simulink model "mrefrobotarm_previous_y_previous_u_previous_ref_cex_3b"  (R2018b)
settings: Solver=FixedStepAuto  StartTime=0.0  StopTime=20  RelTol=1e-3  AbsTol=1e-6
undefined symbols (not defined in the file or in its folder): cc, options
libraries: neural x462, simulink x2
(part 10 of 18)

== system mrefrobotarm_previous_y_previous_u_previous_ref_cex_3b/5000_epoch/Layer 3/Delays 1 ==
  "p{3}" : Inport  PortDimensions=30
      mask Display: e = 0.06;c1 = [120 230 180]/255;c2 = ([120 230 180]+0)/(256+128);c3 = ([120 230 180]+128)/(256+128);patch([0 1 1 0],[0 0 1 1],c1);patch([0 1 1 1-e 1-e 0+e],[0 0 1 1-e 0+e 0+e],c2);patch([0 0 1 1-e 0+e 0+e],[0 1 1 1-e 1-e 0+e],c3);plot([0 1 1 0 0],[0 0 1 1 0]);
  mux : Mux  Inputs=1
      mask Display: e = 0.06;c1 = [120 150 230]/255;c2 = ([120 150 230]+0)/383;c3 = ([120 150 230]+128)/383;patch([0 1 1 0],[0 0 1 1],c1);patch([0 1 1 1-e 1-e 0+e],[0 0 1 1-e 0+e 0+e],c2);patch([0 0 1 1-e 0+e 0+e],[0 1 1 1-e 1-e 0+e],c3);plot([0 1 1 0 0],[0 0 1 1 0]);disp('Mux')
  "pd{3,2}" : Outport
      mask Display: e = 0.06;c1 = [120 230 180]/255;c2 = ([120 230 180]+0)/(256+128);c3 = ([120 230 180]+128)/(256+128);patch([0 1 1 0],[0 0 1 1],c1);patch([0 1 1 1-e 1-e 0+e],[0 0 1 1-e 0+e 0+e],c2);patch([0 0 1 1-e 0+e 0+e],[0 1 1 1-e 1-e 0+e],c3);plot([0 1 1 0 0],[0 0 1 1 0]);
  wires:
  "p{3}"/1 -> mux/1
  mux/1 -> "pd{3,2}"/1

== system mrefrobotarm_previous_y_previous_u_previous_ref_cex_3b/5000_epoch/Layer 3/LW{3,2} ==
  "ad{3,2}" : Inport  PortDimensions=30
      mask Display: e = 0.06;c1 = [120 230 180]/255;c2 = ([120 230 180]+0)/(256+128);c3 = ([120 230 180]+128)/(256+128);patch([0 1 1 0],[0 0 1 1],c1);patch([0 1 1 1-e 1-e 0+e],[0 0 1 1-e 0+e 0+e],c2);patch([0 0 1 1-e 0+e 0+e],[0 1 1 1-e 1-e 0+e],c3);plot([0 1 1 0 0],[0 0 1 1 0]);
  "IW{3,2}(1,:)'" : Constant  Value=[0.07120769791695548411869509664029465056955814361572265625;0.293957514102999251104364475395414046943187713623046875;-0.102217807051302178589224922689027152955532073974609375;-0.4928214954328120622761844060732983052730560302734375;-0.6859335778553450335692787120933644473552703857421875;0.10215887737343372354548165503729251213371753692626953125;0.1810653784287956924448081963419099338352680206298828125;0.278110114235700145446372744117979891598224639892578125;0.165277512488851197058892239510896615684032440185546875;-0.58534311597175092689582243110635317862033843994140625;0.1463336102721248532798625774375977925956249237060546875;-0.134800489251362842768600103227072395384311676025390625;-0.8834099653862776957424784995964728295803070068359375;-0.402877151040579140062192209370550699532032012939453125;-0.9904548377251851665192816653870977461338043212890625;0.07516141105989652959618041450085001997649669647216796875;0.256462278810463517597639793166308663785457611083984375;0.133927541929137861043130897087394259870052337646484375;0.937187293052101910717510691029019653797149658203125;0.344579518523550454300874434920842759311199188232421875;-0.12401331514423587221163103322396636940538883209228515625;-0.7653357924133674661248960546799935400485992431640625;0.6146453163710081657455930326250381767749786376953125;0.2201364801288865080675094532125513069331645965576171875;-0.86449912385295324401823791049537248909473419189453125;-0.543957967972903855269350970047526061534881591796875;0.290966307623606146304240382960415445268154144287109375;0.10258338058370508605321447248570621013641357421875;0.100254156699624397131032083052559755742549896240234375;0.34509165546467002183561589845339767634868621826171875]
      mask Display: e = 0.06;c1 = [120 150 230]/255;c2 = ([120 150 230]+0)/383;c3 = ([120 150 230]+128)/383;patch([0 1 1 0],[0 0 1 1],c1);patch([0 1 1 1-e 1-e 0+e],[0 0 1 1-e 0+e 0+e],c2);patch([0 0 1 1-e 0+e 0+e],[0 1 1 1-e 1-e 0+e],c3);plot([0 1 1 0 0],[0 0 1 1 0]);disp('weights');
  Mux : Mux  Inputs=1
      mask Display: e = 0.06;c1 = [120 150 230]/255;c2 = ([120 150 230]+0)/383;c3 = ([120 150 230]+128)/383;patch([0 1 1 0],[0 0 1 1],c1);patch([0 1 1 1-e 1-e 0+e],[0 0 1 1-e 0+e 0+e],c2);patch([0 0 1 1-e 0+e 0+e],[0 1 1 1-e 1-e 0+e],c3);plot([0 1 1 0 0],[0 0 1 1 0]);disp('Mux');
  dotprod1 : neural/Weight Functions/dotprod
  "lz{3,2}" : Outport
      mask Display: e = 0.06;c1 = [120 230 180]/255;c2 = ([120 230 180]+0)/(256+128);c3 = ([120 230 180]+128)/(256+128);patch([0 1 1 0],[0 0 1 1],c1);patch([0 1 1 1-e 1-e 0+e],[0 0 1 1-e 0+e 0+e],c2);patch([0 0 1 1-e 0+e 0+e],[0 1 1 1-e 1-e 0+e],c3);plot([0 1 1 0 0],[0 0 1 1 0]);
  wires:
  "IW{3,2}(1,:)'"/1 -> dotprod1/1
  "ad{3,2}"/1 -> dotprod1/2
  dotprod1/1 -> Mux/1
  Mux/1 -> "lz{3,2}"/1

== system mrefrobotarm_previous_y_previous_u_previous_ref_cex_3b/cex_m1/Layer 1/Delays 1 ==
  "p{1}" : Inport  PortDimensions=10
      mask Display: e = 0.06;c1 = [120 230 180]/255;c2 = ([120 230 180]+0)/(256+128);c3 = ([120 230 180]+128)/(256+128);patch([0 1 1 0],[0 0 1 1],c1);patch([0 1 1 1-e 1-e 0+e],[0 0 1 1-e 0+e 0+e],c2);patch([0 0 1 1-e 0+e 0+e],[0 1 1 1-e 1-e 0+e],c3);plot([0 1 1 0 0],[0 0 1 1 0]);
  mux : Mux  Inputs=1
      mask Display: e = 0.06;c1 = [120 150 230]/255;c2 = ([120 150 230]+0)/383;c3 = ([120 150 230]+128)/383;patch([0 1 1 0],[0 0 1 1],c1);patch([0 1 1 1-e 1-e 0+e],[0 0 1 1-e 0+e 0+e],c2);patch([0 0 1 1-e 0+e 0+e],[0 1 1 1-e 1-e 0+e],c3);plot([0 1 1 0 0],[0 0 1 1 0]);disp('Mux')
  "pd{1,1}" : Outport
      mask Display: e = 0.06;c1 = [120 230 180]/255;c2 = ([120 230 180]+0)/(256+128);c3 = ([120 230 180]+128)/(256+128);patch([0 1 1 0],[0 0 1 1],c1);patch([0 1 1 1-e 1-e 0+e],[0 0 1 1-e 0+e 0+e],c2);patch([0 0 1 1-e 0+e 0+e],[0 1 1 1-e 1-e 0+e],c3);plot([0 1 1 0 0],[0 0 1 1 0]);
  wires:
  "p{1}"/1 -> mux/1
  mux/1 -> "pd{1,1}"/1

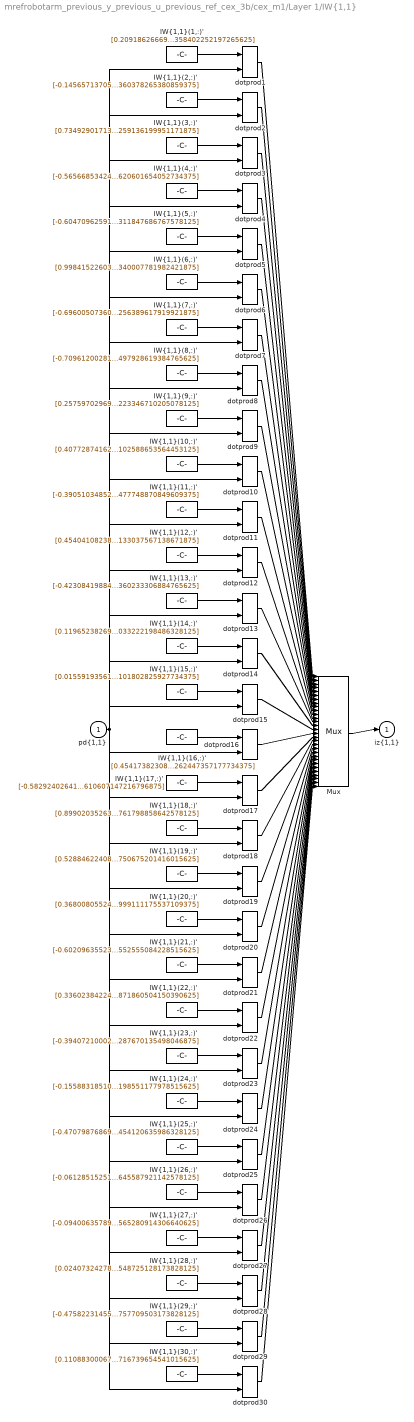
== system mrefrobotarm_previous_y_previous_u_previous_ref_cex_3b/cex_m1/Layer 1/IW{1,1} ==
  "pd{1,1}" : Inport  PortDimensions=10
      mask Display: e = 0.06;c1 = [120 230 180]/255;c2 = ([120 230 180]+0)/(256+128);c3 = ([120 230 180]+128)/(256+128);patch([0 1 1 0],[0 0 1 1],c1);patch([0 1 1 1-e 1-e 0+e],[0 0 1 1-e 0+e 0+e],c2);patch([0 0 1 1-e 0+e 0+e],[0 1 1 1-e 1-e 0+e],c3);plot([0 1 1 0 0],[0 0 1 1 0]);
  "IW{1,1}(1,:)'" : Constant  Value=[0.2091862666929468483889564822675311006605625152587890625;0.55963348740756568844290086417458951473236083984375;0.0245060466286013134418197978448006324470043182373046875;0.2178988291207533400939411194485728628933429718017578125;-0.26749825460170051361075138629530556499958038330078125;0.66511017670048844241392771436949260532855987548828125;-0.89337790569789710115600200879271142184734344482421875;-0.68360390444573138069017659290693700313568115234375;-0.01825482404689289517296657550105010159313678741455078125;-0.88702631490236660827264358886168338358402252197265625]
      mask Display: e = 0.06;c1 = [120 150 230]/255;c2 = ([120 150 230]+0)/383;c3 = ([120 150 230]+128)/383;patch([0 1 1 0],[0 0 1 1],c1);patch([0 1 1 1-e 1-e 0+e],[0 0 1 1-e 0+e 0+e],c2);patch([0 0 1 1-e 0+e 0+e],[0 1 1 1-e 1-e 0+e],c3);plot([0 1 1 0 0],[0 0 1 1 0]);disp('Weights');
  "IW{1,1}(10,:)'" : Constant  Value=[0.407728741626480040149971273422124795615673065185546875;-1.09823873025257778834884447860531508922576904296875;0.29259795109139952185017818919732235372066497802734375;0.345075553219635511315033227219828404486179351806640625;0.6166793772066860856995162976090796291828155517578125;-0.53009927483939034420501457134378142654895782470703125;-0.29346314878497825606729065839317627251148223876953125;0.388864437565445031363964289994328282773494720458984375;-0.022174851916459244194346211997981299646198749542236328125;0.82461100280284871377745048448559828102588653564453125]
      mask Display: e = 0.06;c1 = [120 150 230]/255;c2 = ([120 150 230]+0)/383;c3 = ([120 150 230]+128)/383;patch([0 1 1 0],[0 0 1 1],c1);patch([0 1 1 1-e 1-e 0+e],[0 0 1 1-e 0+e 0+e],c2);patch([0 0 1 1-e 0+e 0+e],[0 1 1 1-e 1-e 0+e],c3);plot([0 1 1 0 0],[0 0 1 1 0]);disp('Weights');
  "IW{1,1}(11,:)'" : Constant  Value=[-0.390510348523106454177167279340210370719432830810546875;0.280930746398683039988242171602905727922916412353515625;0.08856122912073373376617979602087871171534061431884765625;0.0183926105937365184928022898702693055383861064910888671875;-0.08511188285763936212102720446637249551713466644287109375;-1.2933297714879312678704081918112933635711669921875;0.20346443800545410685032265973859466612339019775390625;0.59287238698671185233024516492150723934173583984375;-0.51455352543008781029953979668789543211460113525390625;0.2082980484226676087811114257419831119477748870849609375]
      mask Display: e = 0.06;c1 = [120 150 230]/255;c2 = ([120 150 230]+0)/383;c3 = ([120 150 230]+128)/383;patch([0 1 1 0],[0 0 1 1],c1);patch([0 1 1 1-e 1-e 0+e],[0 0 1 1-e 0+e 0+e],c2);patch([0 0 1 1-e 0+e 0+e],[0 1 1 1-e 1-e 0+e],c3);plot([0 1 1 0 0],[0 0 1 1 0]);disp('Weights');
  "IW{1,1}(12,:)'" : Constant  Value=[0.454041082380829352782569685587077401578426361083984375;-0.108216191956810703356239855565945617854595184326171875;-0.50433758821169483166357849768246524035930633544921875;0.34650587412748390381267427073908038437366485595703125;0.51861097707927428235308298098971135914325714111328125;-0.75606936535445401492694372791447676718235015869140625;-0.474625539848971766954122131210169754922389984130859375;0.062468383097865766429013234528611064888536930084228515625;0.55093241527519953848468503565527498722076416015625;-0.620778109366568298099764433573000133037567138671875]
      mask Display: e = 0.06;c1 = [120 150 230]/255;c2 = ([120 150 230]+0)/383;c3 = ([120 150 230]+128)/383;patch([0 1 1 0],[0 0 1 1],c1);patch([0 1 1 1-e 1-e 0+e],[0 0 1 1-e 0+e 0+e],c2);patch([0 0 1 1-e 0+e 0+e],[0 1 1 1-e 1-e 0+e],c3);plot([0 1 1 0 0],[0 0 1 1 0]);disp('Weights');
  "IW{1,1}(13,:)'" : Constant  Value=[-0.423084198848980796991980923849041573703289031982421875;-0.53304476363188302290296860519447363913059234619140625;-0.565627651828932709321406946401111781597137451171875;0.417830660461573299979676221482804976403713226318359375;0.60632158873281605249161430037929676473140716552734375;0.9207074477285381863822522063856013119220733642578125;-0.95014294107361652041987554184743203222751617431640625;0.0424423038346196934700316205635317601263523101806640625;-0.1643176448134923972599352737233857624232769012451171875;1.0022089026863645333520480562583543360233306884765625]
      mask Display: e = 0.06;c1 = [120 150 230]/255;c2 = ([120 150 230]+0)/383;c3 = ([120 150 230]+128)/383;patch([0 1 1 0],[0 0 1 1],c1);patch([0 1 1 1-e 1-e 0+e],[0 0 1 1-e 0+e 0+e],c2);patch([0 0 1 1-e 0+e 0+e],[0 1 1 1-e 1-e 0+e],c3);plot([0 1 1 0 0],[0 0 1 1 0]);disp('Weights');
  "IW{1,1}(14,:)'" : Constant  Value=[0.1196523826915620869471013065776787698268890380859375;0.203688796664640181521832573707797564566135406494140625;-0.0471376839766617095062173348196665756404399871826171875;0.474187802455269091783662815942079760134220123291015625;-1.019539841234085475463189141009934246540069580078125;0.31052365757284672298510486143641173839569091796875;-0.7583308622335831472582867718301713466644287109375;0.2650487385605939660848662242642603814601898193359375;0.05457125001518541018707963985434616915881633758544921875;-0.0952582112585181051134242125044693239033222198486328125]
      mask Display: e = 0.06;c1 = [120 150 230]/255;c2 = ([120 150 230]+0)/383;c3 = ([120 150 230]+128)/383;patch([0 1 1 0],[0 0 1 1],c1);patch([0 1 1 1-e 1-e 0+e],[0 0 1 1-e 0+e 0+e],c2);patch([0 0 1 1-e 0+e 0+e],[0 1 1 1-e 1-e 0+e],c3);plot([0 1 1 0 0],[0 0 1 1 0]);disp('Weights');
  "IW{1,1}(15,:)'" : Constant  Value=[0.0155919356143503391731730545188838732428848743438720703125;0.269803619589356113994682573320460505783557891845703125;0.147051842439241242654901498099206946790218353271484375;-0.7745868105897117938951623727916739881038665771484375;1.2903168482513975856562638000468723475933074951171875;-0.4201312277855315802099767097388394176959991455078125;-0.226047840789400933392272463606786914169788360595703125;-0.72869256085332534400578197164577431976795196533203125;-0.40668314497398128093408331551472656428813934326171875;-0.74033295636701035302706941365613602101802825927734375]
      mask Display: e = 0.06;c1 = [120 150 230]/255;c2 = ([120 150 230]+0)/383;c3 = ([120 150 230]+128)/383;patch([0 1 1 0],[0 0 1 1],c1);patch([0 1 1 1-e 1-e 0+e],[0 0 1 1-e 0+e 0+e],c2);patch([0 0 1 1-e 0+e 0+e],[0 1 1 1-e 1-e 0+e],c3);plot([0 1 1 0 0],[0 0 1 1 0]);disp('Weights');
  "IW{1,1}(16,:)'" : Constant  Value=[0.454173823086521932790304845184436999261379241943359375;-0.800364086576109468040840511093847453594207763671875;0.280125159478748997354813354832003824412822723388671875;-0.8182209528732153902552681756787933409214019775390625;1.8090173847658237438196238144882954657077789306640625;0.5022417744867786471019144300953485071659088134765625;-1.169078109472902138321614984306506812572479248046875;-0.5998812716593977523160674536484293639659881591796875;-0.0400917281417088322559294510938343591988086700439453125;0.331029591208813422920087532475008629262447357177734375]
      mask Display: e = 0.06;c1 = [120 150 230]/255;c2 = ([120 150 230]+0)/383;c3 = ([120 150 230]+128)/383;patch([0 1 1 0],[0 0 1 1],c1);patch([0 1 1 1-e 1-e 0+e],[0 0 1 1-e 0+e 0+e],c2);patch([0 0 1 1-e 0+e 0+e],[0 1 1 1-e 1-e 0+e],c3);plot([0 1 1 0 0],[0 0 1 1 0]);disp('Weights');
  "IW{1,1}(17,:)'" : Constant  Value=[-0.5829240264146486882879116819822229444980621337890625;0.98504904866951614739178921809070743620395660400390625;-0.2542168950231253887750426656566560268402099609375;0.509425718623048862099267353187315165996551513671875;0.71815029183283496383438659904641099274158477783203125;-0.97456899966675691882045384772936813533306121826171875;-0.1697229391253351205026689285659813322126865386962890625;0.1636748206886007028781904182324069552123546600341796875;0.255098819940770826786291536336648277938365936279296875;-0.5024198673275594995146775545435957610607147216796875]
      mask Display: e = 0.06;c1 = [120 150 230]/255;c2 = ([120 150 230]+0)/383;c3 = ([120 150 230]+128)/383;patch([0 1 1 0],[0 0 1 1],c1);patch([0 1 1 1-e 1-e 0+e],[0 0 1 1-e 0+e 0+e],c2);patch([0 0 1 1-e 0+e 0+e],[0 1 1 1-e 1-e 0+e],c3);plot([0 1 1 0 0],[0 0 1 1 0]);disp('Weights');
  "IW{1,1}(18,:)'" : Constant  Value=[0.8990203526391773447556943210656754672527313232421875;-0.471686438787703832264952552577597089111804962158203125;-0.892914200230652710388312698341906070709228515625;-0.07007749122282362630453889096315833739936351776123046875;0.1677092178341874906255526411769096739590167999267578125;0.279705943970333492654134488475392572581768035888671875;0.1259915830780845846792459497009986080229282379150390625;-0.6503287762770748603458059733384288847446441650390625;-0.6518112623153899942707312220591120421886444091796875;-0.56845180521082661062592933376436121761798858642578125]
      mask Display: e = 0.06;c1 = [120 150 230]/255;c2 = ([120 150 230]+0)/383;c3 = ([120 150 230]+128)/383;patch([0 1 1 0],[0 0 1 1],c1);patch([0 1 1 1-e 1-e 0+e],[0 0 1 1-e 0+e 0+e],c2);patch([0 0 1 1-e 0+e 0+e],[0 1 1 1-e 1-e 0+e],c3);plot([0 1 1 0 0],[0 0 1 1 0]);disp('Weights');
  "IW{1,1}(19,:)'" : Constant  Value=[0.52884622408495352008372947238967753946781158447265625;0.34089759980611511469561492049251683056354522705078125;-0.448295411265493048968977518597966991364955902099609375;0.7316745664736530319061103000422008335590362548828125;0.01119555977979982096248701139984405017457902431488037109375;-0.87063334773666412047532503493130207061767578125;0.7710191192510136293236655546934343874454498291015625;0.70429711176034748287833053836948238313198089599609375;0.53710793489006924961159938902710564434528350830078125;-0.54623479056526580421859762282110750675201416015625]
      mask Display: e = 0.06;c1 = [120 150 230]/255;c2 = ([120 150 230]+0)/383;c3 = ([120 150 230]+128)/383;patch([0 1 1 0],[0 0 1 1],c1);patch([0 1 1 1-e 1-e 0+e],[0 0 1 1-e 0+e 0+e],c2);patch([0 0 1 1-e 0+e 0+e],[0 1 1 1-e 1-e 0+e],c3);plot([0 1 1 0 0],[0 0 1 1 0]);disp('Weights');
  "IW{1,1}(2,:)'" : Constant  Value=[-0.14565713705002547584399508195929229259490966796875;0.92722440151880702874365169918746687471866607666015625;-0.58041816336865037495584829230210743844509124755859375;0.327140195131600031164254005489055998623371124267578125;-0.929859979711404438518229653709568083286285400390625;-0.74872830114199062645496951517998240888118743896484375;0.385940683264537398589055783304502256214618682861328125;0.6107778553311418168192403754801489412784576416015625;0.75481290789782995442891433413024060428142547607421875;-0.235879183916507084717295583686791360378265380859375]
      mask Display: e = 0.06;c1 = [120 150 230]/255;c2 = ([120 150 230]+0)/383;c3 = ([120 150 230]+128)/383;patch([0 1 1 0],[0 0 1 1],c1);patch([0 1 1 1-e 1-e 0+e],[0 0 1 1-e 0+e 0+e],c2);patch([0 0 1 1-e 0+e 0+e],[0 1 1 1-e 1-e 0+e],c3);plot([0 1 1 0 0],[0 0 1 1 0]);disp('Weights');
  "IW{1,1}(20,:)'" : Constant  Value=[0.368008055243381371202104901385609991848468780517578125;-0.002192585139888168256627754004739472293294966220855712890625;0.0563330526990998559089263153509818948805332183837890625;0.352091098525261270157926674073678441345691680908203125;0.385736390538022166918352695574867539107799530029296875;-0.247630614263226467297585031701601110398769378662109375;0.58477909697959418178214718864182941615581512451171875;0.1562187305741310205942085076458170078694820404052734375;0.82360238974781430076888000257895328104496002197265625;-0.476230943299036757476727643734193406999111175537109375]
      mask Display: e = 0.06;c1 = [120 150 230]/255;c2 = ([120 150 230]+0)/383;c3 = ([120 150 230]+128)/383;patch([0 1 1 0],[0 0 1 1],c1);patch([0 1 1 1-e 1-e 0+e],[0 0 1 1-e 0+e 0+e],c2);patch([0 0 1 1-e 0+e 0+e],[0 1 1 1-e 1-e 0+e],c3);plot([0 1 1 0 0],[0 0 1 1 0]);disp('Weights');
  "IW{1,1}(21,:)'" : Constant  Value=[-0.60209635523566762405067720465012826025485992431640625;-0.0716463435268997195226603480477933771908283233642578125;0.271658003646719325985259274602867662906646728515625;-0.5095289852754951720470444342936389148235321044921875;0.15508802660567211351150262998999096453189849853515625;-0.400285938688359710369013555464334785938262939453125;0.147605255136038504559792272630147635936737060546875;-0.0248094629809944879073047019346631714142858982086181640625;-1.0605743434036065675485360770835541188716888427734375;0.69405662206880069931003163219429552555084228515625]
      mask Display: e = 0.06;c1 = [120 150 230]/255;c2 = ([120 150 230]+0)/383;c3 = ([120 150 230]+128)/383;patch([0 1 1 0],[0 0 1 1],c1);patch([0 1 1 1-e 1-e 0+e],[0 0 1 1-e 0+e 0+e],c2);patch([0 0 1 1-e 0+e 0+e],[0 1 1 1-e 1-e 0+e],c3);plot([0 1 1 0 0],[0 0 1 1 0]);disp('Weights');
  "IW{1,1}(22,:)'" : Constant  Value=[0.33602384224934456202760202359058894217014312744140625;0.316854130288579616259170279590762220323085784912109375;-0.37857291065639475657889079229789786040782928466796875;0.85810737036911899355828836633008904755115509033203125;-1.04134819912401699326665038825012743473052978515625;0.348267620019931722907813309575431048870086669921875;0.68524259659312536374642377268173731863498687744140625;0.68116189574731322853295978347887285053730010986328125;0.053809239235190174654999140102518140338361263275146484375;0.071470638811097553233508961056941188871860504150390625]
      mask Display: e = 0.06;c1 = [120 150 230]/255;c2 = ([120 150 230]+0)/383;c3 = ([120 150 230]+128)/383;patch([0 1 1 0],[0 0 1 1],c1);patch([0 1 1 1-e 1-e 0+e],[0 0 1 1-e 0+e 0+e],c2);patch([0 0 1 1-e 0+e 0+e],[0 1 1 1-e 1-e 0+e],c3);plot([0 1 1 0 0],[0 0 1 1 0]);disp('Weights');
  "IW{1,1}(23,:)'" : Constant  Value=[-0.394072100026185534460410053725354373455047607421875;1.11211173361084636468376629636622965335845947265625;-0.320213097632206455944725576046039350330829620361328125;0.50688355043374588859705909271724522113800048828125;-0.0849486697110029276291953692634706385433673858642578125;-0.96291306803094289801236982384580187499523162841796875;-0.377668560200759617639931775556760840117931365966796875;0.0946944889176795923102503138579777441918849945068359375;-0.32170494180800834893574347006506286561489105224609375;-0.5240786394310272822139040727051906287670135498046875]
      mask Display: e = 0.06;c1 = [120 150 230]/255;c2 = ([120 150 230]+0)/383;c3 = ([120 150 230]+128)/383;patch([0 1 1 0],[0 0 1 1],c1);patch([0 1 1 1-e 1-e 0+e],[0 0 1 1-e 0+e 0+e],c2);patch([0 0 1 1-e 0+e 0+e],[0 1 1 1-e 1-e 0+e],c3);plot([0 1 1 0 0],[0 0 1 1 0]);disp('Weights');
  "IW{1,1}(24,:)'" : Constant  Value=[-0.1558831851007405067122135733370669186115264892578125;0.844094882972143079058469083975069224834442138671875;-0.162691690832094337793023441918194293975830078125;0.016237577929413653243795323533049668185412883758544921875;-1.1894624225200374212363385595381259918212890625;0.82329478893758312185724435039446689188480377197265625;0.1589582061303255466899742032182984985411167144775390625;0.6871248504549163360621832907781936228275299072265625;0.58317539415476515873848484261543489992618560791015625;0.74057525253661238284763612682581879198551177978515625]
      mask Display: e = 0.06;c1 = [120 150 230]/255;c2 = ([120 150 230]+0)/383;c3 = ([120 150 230]+128)/383;patch([0 1 1 0],[0 0 1 1],c1);patch([0 1 1 1-e 1-e 0+e],[0 0 1 1-e 0+e 0+e],c2);patch([0 0 1 1-e 0+e 0+e],[0 1 1 1-e 1-e 0+e],c3);plot([0 1 1 0 0],[0 0 1 1 0]);disp('Weights');
  "IW{1,1}(25,:)'" : Constant  Value=[-0.470798768696179925630218576770857907831668853759765625;0.5088878241581531458592735361889936029911041259765625;-0.611957297078266737599960833904333412647247314453125;-0.2312082540432938981833643765639862976968288421630859375;0.83570652856447136258566388278268277645111083984375;-0.118154714584164877155814110665232874453067779541015625;0.35551510319171286678141541415243409574031829833984375;-0.8469436595621215868590070385835133492946624755859375;-0.59937255562654867535599123584688641130924224853515625;0.66725706794129735488496635298361070454120635986328125]
      mask Display: e = 0.06;c1 = [120 150 230]/255;c2 = ([120 150 230]+0)/383;c3 = ([120 150 230]+128)/383;patch([0 1 1 0],[0 0 1 1],c1);patch([0 1 1 1-e 1-e 0+e],[0 0 1 1-e 0+e 0+e],c2);patch([0 0 1 1-e 0+e 0+e],[0 1 1 1-e 1-e 0+e],c3);plot([0 1 1 0 0],[0 0 1 1 0]);disp('Weights');
  "IW{1,1}(26,:)'" : Constant  Value=[-0.061285152510976374784501530257330159656703472137451171875;-0.347078272120007691459164789193891920149326324462890625;0.79386039204182001771670229572919197380542755126953125;-0.1920622851114592577470574497056077234447002410888671875;-0.267201831261956013197078618759405799210071563720703125;0.7955336654175482191675428111921064555644989013671875;-0.52745915842468471534942864309414289891719818115234375;-0.451184299445789249727312153481761924922466278076171875;-0.70192132144373264868164596919086761772632598876953125;-0.01597233306397490004702177657236461527645587921142578125]
      mask Display: e = 0.06;c1 = [120 150 230]/255;c2 = ([120 150 230]+0)/383;c3 = ([120 150 230]+128)/383;patch([0 1 1 0],[0 0 1 1],c1);patch([0 1 1 1-e 1-e 0+e],[0 0 1 1-e 0+e 0+e],c2);patch([0 0 1 1-e 0+e 0+e],[0 1 1 1-e 1-e 0+e],c3);plot([0 1 1 0 0],[0 0 1 1 0]);disp('Weights');
  "IW{1,1}(27,:)'" : Constant  Value=[-0.094006357895163372706548443602514453232288360595703125;0.50258758717796070403238672952284105122089385986328125;-0.3250885797258644682727890540263615548610687255859375;0.6097656985874697621596851604408584535121917724609375;-0.768193443515825524769979892880655825138092041015625;-0.26588773231290752097066842907224781811237335205078125;0.2411467561153750882585455883599934168159961700439453125;-0.2118771976848636551249427384391310624778270721435546875;0.8123245037821018588175547847640700638294219970703125;-0.77592928965660379336810592576512135565280914306640625]
      mask Display: e = 0.06;c1 = [120 150 230]/255;c2 = ([120 150 230]+0)/383;c3 = ([120 150 230]+128)/383;patch([0 1 1 0],[0 0 1 1],c1);patch([0 1 1 1-e 1-e 0+e],[0 0 1 1-e 0+e 0+e],c2);patch([0 0 1 1-e 0+e 0+e],[0 1 1 1-e 1-e 0+e],c3);plot([0 1 1 0 0],[0 0 1 1 0]);disp('Weights');
  "IW{1,1}(28,:)'" : Constant  Value=[0.0240732427837186298280602869681388256140053272247314453125;0.28489018584777625608950302193989045917987823486328125;0.0080037004159878820386264663966358057223260402679443359375;0.41812597240847093615911944652907550334930419921875;-0.3610111948086041078198604736826382577419281005859375;0.75828857348877398703024255155469290912151336669921875;-0.89565724853786032877422940146061591804027557373046875;-0.313002141447430382026340112133766524493694305419921875;0.56933330116754088390251808959874324500560760498046875;0.495197397438050856965929824582417495548725128173828125]
      mask Display: e = 0.06;c1 = [120 150 230]/255;c2 = ([120 150 230]+0)/383;c3 = ([120 150 230]+128)/383;patch([0 1 1 0],[0 0 1 1],c1);patch([0 1 1 1-e 1-e 0+e],[0 0 1 1-e 0+e 0+e],c2);patch([0 0 1 1-e 0+e 0+e],[0 1 1 1-e 1-e 0+e],c3);plot([0 1 1 0 0],[0 0 1 1 0]);disp('Weights');
  "IW{1,1}(29,:)'" : Constant  Value=[-0.475822314554792347163214571992284618318080902099609375;-0.40778440343508126630922561162151396274566650390625;0.1290514951888164507654011003978666849434375762939453125;0.54678823531480691411132966095465235412120819091796875;1.033496587893427243187716157990507781505584716796875;-0.0932158538272811754143987172938068397343158721923828125;0.321067421729369251170993493360583670437335968017578125;-0.49566110110721961490298781427554786205291748046875;-0.62601974388640335700273453767294995486736297607421875;0.78146921983346928630709271601517684757709503173828125]
      mask Display: e = 0.06;c1 = [120 150 230]/255;c2 = ([120 150 230]+0)/383;c3 = ([120 150 230]+128)/383;patch([0 1 1 0],[0 0 1 1],c1);patch([0 1 1 1-e 1-e 0+e],[0 0 1 1-e 0+e 0+e],c2);patch([0 0 1 1-e 0+e 0+e],[0 1 1 1-e 1-e 0+e],c3);plot([0 1 1 0 0],[0 0 1 1 0]);disp('Weights');
  "IW{1,1}(3,:)'" : Constant  Value=[0.73492901713567870825016825619968585669994354248046875;-0.12445375499860412971120382508161128498613834381103515625;-0.188614430554673695450418335894937627017498016357421875;0.528323809103511177198697623680345714092254638671875;-0.77072921666130145279538510294514708220958709716796875;-0.46789224997181488863162712732446379959583282470703125;-0.60091732188756719068578604492358863353729248046875;0.212446317890346014767288806979195214807987213134765625;0.4884554484686869368914585720631293952465057373046875;0.3759027830975707473726288299076259136199951171875]
      mask Display: e = 0.06;c1 = [120 150 230]/255;c2 = ([120 150 230]+0)/383;c3 = ([120 150 230]+128)/383;patch([0 1 1 0],[0 0 1 1],c1);patch([0 1 1 1-e 1-e 0+e],[0 0 1 1-e 0+e 0+e],c2);patch([0 0 1 1-e 0+e 0+e],[0 1 1 1-e 1-e 0+e],c3);plot([0 1 1 0 0],[0 0 1 1 0]);disp('Weights');
  "IW{1,1}(30,:)'" : Constant  Value=[0.1108830006720775418482816121468204073607921600341796875;0.27597424138404746951636070662061683833599090576171875;0.07237656155913220479281022790019051171839237213134765625;-0.6718780995107562770130016360781155526638031005859375;0.26512327461840523579184036861988715827465057373046875;0.022014613654137003828648033731951727531850337982177734375;-0.460158949503963354832336563049466349184513092041015625;0.8965832665283499647301823642919771373271942138671875;1.1260509320261788968053906501154415309429168701171875;0.87081583998190181805654219715506769716739654541015625]
      mask Display: e = 0.06;c1 = [120 150 230]/255;c2 = ([120 150 230]+0)/383;c3 = ([120 150 230]+128)/383;patch([0 1 1 0],[0 0 1 1],c1);patch([0 1 1 1-e 1-e 0+e],[0 0 1 1-e 0+e 0+e],c2);patch([0 0 1 1-e 0+e 0+e],[0 1 1 1-e 1-e 0+e],c3);plot([0 1 1 0 0],[0 0 1 1 0]);disp('Weights');
  "IW{1,1}(4,:)'" : Constant  Value=[-0.56566853424337215638928455518907867372035980224609375;0.419895057554090789242451364771113730967044830322265625;0.337028449185336087534636817508726380765438079833984375;-0.16918513399525958451619089828454889357089996337890625;-0.17183457369647625601061236011446453630924224853515625;0.94252173582833742582209879401489160954952239990234375;0.457691037022962932123704149489640258252620697021484375;-0.82207247901612834350970615560072474181652069091796875;0.86551592689290057780482356974971480667591094970703125;-1.0045585920783446365334157235338352620601654052734375]
      mask Display: e = 0.06;c1 = [120 150 230]/255;c2 = ([120 150 230]+0)/383;c3 = ([120 150 230]+128)/383;patch([0 1 1 0],[0 0 1 1],c1);patch([0 1 1 1-e 1-e 0+e],[0 0 1 1-e 0+e 0+e],c2);patch([0 0 1 1-e 0+e 0+e],[0 1 1 1-e 1-e 0+e],c3);plot([0 1 1 0 0],[0 0 1 1 0]);disp('Weights');
  "IW{1,1}(5,:)'" : Constant  Value=[-0.60470962591841492805855295955552719533443450927734375;-0.262214275897764803602285610395483672618865966796875;0.427621773582947450886848628215375356376171112060546875;-0.649172400280064731958873380790464580059051513671875;0.596218418344656608809373210533522069454193115234375;0.9524625511839566183169836222077719867229461669921875;-0.03585632731938619144340663069669972173869609832763671875;-0.129445611126129456192046518481220118701457977294921875;-0.5202595903826481293918959636357612907886505126953125;0.8612686570422234400012939659063704311847686767578125]
      mask Display: e = 0.06;c1 = [120 150 230]/255;c2 = ([120 150 230]+0)/383;c3 = ([120 150 230]+128)/383;patch([0 1 1 0],[0 0 1 1],c1);patch([0 1 1 1-e 1-e 0+e],[0 0 1 1-e 0+e 0+e],c2);patch([0 0 1 1-e 0+e 0+e],[0 1 1 1-e 1-e 0+e],c3);plot([0 1 1 0 0],[0 0 1 1 0]);disp('Weights');
  "IW{1,1}(6,:)'" : Constant  Value=[0.99841522603030596894058135148952715098857879638671875;-0.78257941390648866342161227294127456843852996826171875;0.154609767416673815620953291727346368134021759033203125;-0.96857238723604621721818830337724648416042327880859375;0.52274988909580366591711708679213188588619232177734375;-0.1616261634770763955248895626937155611813068389892578125;-0.3723828792949521737654094977187924087047576904296875;0.0923787881738797889141778796329163014888763427734375;-0.6826357475149975595485329904477111995220184326171875;0.63696150487462765976687251168186776340007781982421875]
      mask Display: e = 0.06;c1 = [120 150 230]/255;c2 = ([120 150 230]+0)/383;c3 = ([120 150 230]+128)/383;patch([0 1 1 0],[0 0 1 1],c1);patch([0 1 1 1-e 1-e 0+e],[0 0 1 1-e 0+e 0+e],c2);patch([0 0 1 1-e 0+e 0+e],[0 1 1 1-e 1-e 0+e],c3);plot([0 1 1 0 0],[0 0 1 1 0]);disp('Weights');
  "IW{1,1}(7,:)'" : Constant  Value=[-0.696005073606627444604555421392433345317840576171875;-0.8958318511098408709614204781246371567249298095703125;1.1102935209340276667688840461778454482555389404296875;-0.056568430059580732116586432312033139169216156005859375;-0.413492806098580356621852160969865508377552032470703125;0.54102709125570525028336987816146574914455413818359375;0.8508470430380299376338371075689792633056640625;0.11510239975819523683409073555594659410417079925537109375;0.3363906297741070527962392588960938155651092529296875;0.175524857553401580911867085887934081256389617919921875]
      mask Display: e = 0.06;c1 = [120 150 230]/255;c2 = ([120 150 230]+0)/383;c3 = ([120 150 230]+128)/383;patch([0 1 1 0],[0 0 1 1],c1);patch([0 1 1 1-e 1-e 0+e],[0 0 1 1-e 0+e 0+e],c2);patch([0 0 1 1-e 0+e 0+e],[0 1 1 1-e 1-e 0+e],c3);plot([0 1 1 0 0],[0 0 1 1 0]);disp('Weights');
  "IW{1,1}(8,:)'" : Constant  Value=[-0.70961200281083158802886146077071316540241241455078125;0.3130387996628538616050718701444566249847412109375;0.246047662351558837912079980014823377132415771484375;0.284909466821933410329847902175970375537872314453125;0.8315675869131216035867737446096725761890411376953125;0.129241580863567406822767225094139575958251953125;-0.85964958884306519326656825796817429363727569580078125;0.27573677713937472244509763186215423047542572021484375;-0.73426514156710409597650368596077896654605865478515625;-0.81183015488473719845075038392678834497928619384765625]
      mask Display: e = 0.06;c1 = [120 150 230]/255;c2 = ([120 150 230]+0)/383;c3 = ([120 150 230]+128)/383;patch([0 1 1 0],[0 0 1 1],c1);patch([0 1 1 1-e 1-e 0+e],[0 0 1 1-e 0+e 0+e],c2);patch([0 0 1 1-e 0+e 0+e],[0 1 1 1-e 1-e 0+e],c3);plot([0 1 1 0 0],[0 0 1 1 0]);disp('Weights');
  "IW{1,1}(9,:)'" : Constant  Value=[0.257597029691410128737771856322069652378559112548828125;-0.10907000246296470746809603724614134989678859710693359375;-1.12896069637251361683638606336899101734161376953125;0.5665098273955979646387959292042069137096405029296875;-0.233567852824058952432295654944027774035930633544921875;-0.3696298142221976501531344183604232966899871826171875;-0.2304723170385860331332850137187051586806774139404296875;-0.2340417687308379568467131548459292389452457427978515625;-0.65822939402727431712492034421302378177642822265625;0.1889727445051719023627612159543787129223346710205078125]
      mask Display: e = 0.06;c1 = [120 150 230]/255;c2 = ([120 150 230]+0)/383;c3 = ([120 150 230]+128)/383;patch([0 1 1 0],[0 0 1 1],c1);patch([0 1 1 1-e 1-e 0+e],[0 0 1 1-e 0+e 0+e],c2);patch([0 0 1 1-e 0+e 0+e],[0 1 1 1-e 1-e 0+e],c3);plot([0 1 1 0 0],[0 0 1 1 0]);disp('Weights');
  Mux : Mux  Inputs=30
      mask Display: e = 0.06;c1 = [120 150 230]/255;c2 = ([120 150 230]+0)/383;c3 = ([120 150 230]+128)/383;patch([0 1 1 0],[0 0 1 1],c1);patch([0 1 1 1-e 1-e 0+e],[0 0 1 1-e 0+e 0+e],c2);patch([0 0 1 1-e 0+e 0+e],[0 1 1 1-e 1-e 0+e],c3);plot([0 1 1 0 0],[0 0 1 1 0]);disp('Mux');
  dotprod{1..30} (30 alike) : neural/Weight Functions/dotprod
  "iz{1,1}" : Outport
      mask Display: e = 0.06;c1 = [120 230 180]/255;c2 = ([120 230 180]+0)/(256+128);c3 = ([120 230 180]+128)/(256+128);patch([0 1 1 0],[0 0 1 1],c1);patch([0 1 1 1-e 1-e 0+e],[0 0 1 1-e 0+e 0+e],c2);patch([0 0 1 1-e 0+e 0+e],[0 1 1 1-e 1-e 0+e],c3);plot([0 1 1 0 0],[0 0 1 1 0]);
  wires:
  "IW{1,1}(1,:)'"/1 -> dotprod1/1
  "pd{1,1}"/1 -> dotprod1/2, dotprod2/2, dotprod3/2, dotprod4/2, dotprod5/2, dotprod6/2, dotprod7/2, dotprod8/2, dotprod9/2, dotprod10/2, dotprod11/2, dotprod12/2, dotprod13/2, dotprod14/2, dotprod15/2, dotprod16/2, dotprod17/2, dotprod18/2, dotprod19/2, dotprod20/2, dotprod21/2, dotprod22/2, dotprod23/2, dotprod24/2, dotprod25/2, dotprod26/2, dotprod27/2, dotprod28/2, dotprod29/2, dotprod30/2
  dotprod1/1 -> Mux/1
  "IW{1,1}(2,:)'"/1 -> dotprod2/1
  dotprod2/1 -> Mux/2
  "IW{1,1}(3,:)'"/1 -> dotprod3/1
  dotprod3/1 -> Mux/3
  "IW{1,1}(4,:)'"/1 -> dotprod4/1
  dotprod4/1 -> Mux/4
  "IW{1,1}(5,:)'"/1 -> dotprod5/1
  dotprod5/1 -> Mux/5
  "IW{1,1}(6,:)'"/1 -> dotprod6/1
  dotprod6/1 -> Mux/6
  "IW{1,1}(7,:)'"/1 -> dotprod7/1
  dotprod7/1 -> Mux/7
  "IW{1,1}(8,:)'"/1 -> dotprod8/1
  dotprod8/1 -> Mux/8
  "IW{1,1}(9,:)'"/1 -> dotprod9/1
  dotprod9/1 -> Mux/9
  "IW{1,1}(10,:)'"/1 -> dotprod10/1
  dotprod10/1 -> Mux/10
  "IW{1,1}(11,:)'"/1 -> dotprod11/1
  dotprod11/1 -> Mux/11
  "IW{1,1}(12,:)'"/1 -> dotprod12/1
  dotprod12/1 -> Mux/12
  "IW{1,1}(13,:)'"/1 -> dotprod13/1
  dotprod13/1 -> Mux/13
  "IW{1,1}(14,:)'"/1 -> dotprod14/1
  dotprod14/1 -> Mux/14
  "IW{1,1}(15,:)'"/1 -> dotprod15/1
  dotprod15/1 -> Mux/15
  "IW{1,1}(16,:)'"/1 -> dotprod16/1
  dotprod16/1 -> Mux/16
  "IW{1,1}(17,:)'"/1 -> dotprod17/1
  dotprod17/1 -> Mux/17
  "IW{1,1}(18,:)'"/1 -> dotprod18/1
  dotprod18/1 -> Mux/18
  "IW{1,1}(19,:)'"/1 -> dotprod19/1
  dotprod19/1 -> Mux/19
  "IW{1,1}(20,:)'"/1 -> dotprod20/1
  dotprod20/1 -> Mux/20
  "IW{1,1}(21,:)'"/1 -> dotprod21/1
  dotprod21/1 -> Mux/21
  "IW{1,1}(22,:)'"/1 -> dotprod22/1
  dotprod22/1 -> Mux/22
  "IW{1,1}(23,:)'"/1 -> dotprod23/1
  dotprod23/1 -> Mux/23
  "IW{1,1}(24,:)'"/1 -> dotprod24/1
  dotprod24/1 -> Mux/24
  "IW{1,1}(25,:)'"/1 -> dotprod25/1
  dotprod25/1 -> Mux/25
  "IW{1,1}(26,:)'"/1 -> dotprod26/1
  dotprod26/1 -> Mux/26
  "IW{1,1}(27,:)'"/1 -> dotprod27/1
  dotprod27/1 -> Mux/27
  "IW{1,1}(28,:)'"/1 -> dotprod28/1
  dotprod28/1 -> Mux/28
  "IW{1,1}(29,:)'"/1 -> dotprod29/1
  dotprod29/1 -> Mux/29
  "IW{1,1}(30,:)'"/1 -> dotprod30/1
  dotprod30/1 -> Mux/30
  Mux/1 -> "iz{1,1}"/1

== system mrefrobotarm_previous_y_previous_u_previous_ref_cex_3b/cex_m1/Layer 2/Delays 1 ==
  "p{2}" : Inport  PortDimensions=30
      mask Display: e = 0.06;c1 = [120 230 180]/255;c2 = ([120 230 180]+0)/(256+128);c3 = ([120 230 180]+128)/(256+128);patch([0 1 1 0],[0 0 1 1],c1);patch([0 1 1 1-e 1-e 0+e],[0 0 1 1-e 0+e 0+e],c2);patch([0 0 1 1-e 0+e 0+e],[0 1 1 1-e 1-e 0+e],c3);plot([0 1 1 0 0],[0 0 1 1 0]);
  mux : Mux  Inputs=1
      mask Display: e = 0.06;c1 = [120 150 230]/255;c2 = ([120 150 230]+0)/383;c3 = ([120 150 230]+128)/383;patch([0 1 1 0],[0 0 1 1],c1);patch([0 1 1 1-e 1-e 0+e],[0 0 1 1-e 0+e 0+e],c2);patch([0 0 1 1-e 0+e 0+e],[0 1 1 1-e 1-e 0+e],c3);plot([0 1 1 0 0],[0 0 1 1 0]);disp('Mux')
  "pd{2,1}" : Outport
      mask Display: e = 0.06;c1 = [120 230 180]/255;c2 = ([120 230 180]+0)/(256+128);c3 = ([120 230 180]+128)/(256+128);patch([0 1 1 0],[0 0 1 1],c1);patch([0 1 1 1-e 1-e 0+e],[0 0 1 1-e 0+e 0+e],c2);patch([0 0 1 1-e 0+e 0+e],[0 1 1 1-e 1-e 0+e],c3);plot([0 1 1 0 0],[0 0 1 1 0]);
  wires:
  "p{2}"/1 -> mux/1
  mux/1 -> "pd{2,1}"/1
